simulink model "plant2016_cybership_detectabl_switching_bumplessExperiment"  (R2015b)
settings: Solver=VariableStepAuto  SolverMode=SingleTasking  StartTime=0.0  StopTime=150  FixedStep=.01  RelTol=1e-3  AbsTol=1e-6
StartFcn:
  | %plot_Contr_index('open')
libraries: simulink x9
(part 1 of 2)
CloseFcn:
  | ;slview('closediagram',bdroot);
settings Model: ExtModeTrigMode=oneshot  ExtModeArmWhenConnect=off  Creator=mjun  LastModifiedBy=TordFO
settings DataIOCC: LimitDataPoints=off  SaveFormat=Array  SignalLoggingSaveFormat=ModelDataLogs  SaveOutput=off  SaveTime=off
settings OptimizationCC: BlockReduction=off  BooleanDataType=off
settings DebuggingCC: SaveWithParameterizedLinksMsg=none  UnderspecifiedInitializationDetection=Classic  MergeDetectMultiDrivingBlocksExec=none  SignalResolutionControl=TryResolveAllWithWarning  MultiTaskDSMMsg=warning  MultiTaskCondExecSysMsg=none
settings HardwareCC: ProdBitPerPointer=32  ProdLargestAtomicFloat=None  ProdIntDivRoundTo=Undefined  ProdEndianess=Unspecified  ProdWordSize=32  ProdHWDeviceType=32-bit Generic  TargetUnknown=on
settings RTWCC: TemplateMakefile=grt_unix.tmf
settings GRTTargetCC: GeneratePreprocessorConditionals=Disable all  CombineOutputUpdateFcns=off  GRTInterface=on
settings ConfigComp: CovModelRefEnable=Off  CovSFcnEnable=off

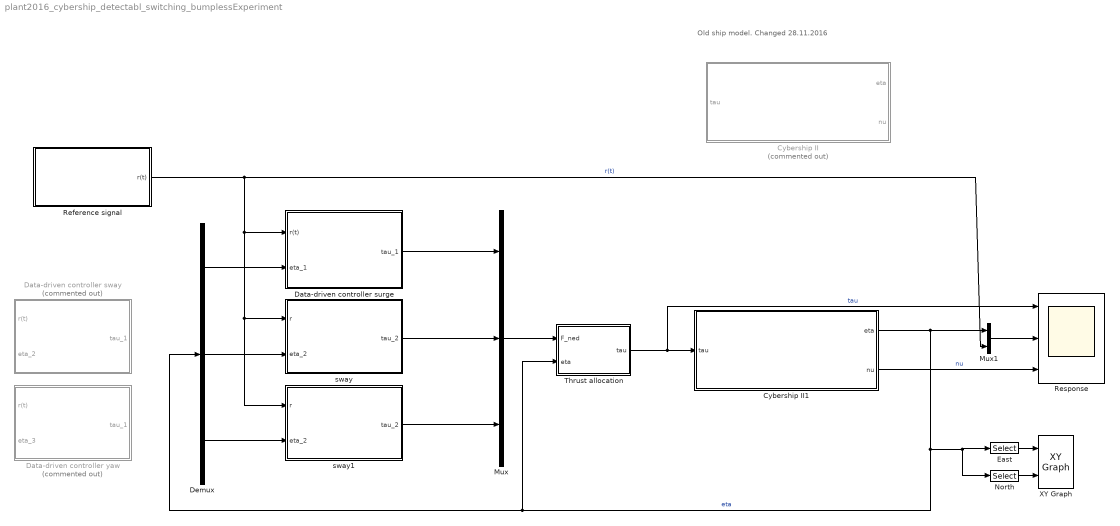
== system plant2016_cybership_detectabl_switching_bumplessExperiment ==
  note: Old ship model. Changed 28.11.2016
  Cybership II : Subsystem  Commented=on  mask{eta_0=[1;2;20*pi/180], nu_0=[0;0;0], first_order_waves_on_off=off, wind_on_off=off, surge_only=off}
      mask prompts: eta_0 "Position initial state"; nu_0 "Velocity initial state"; first_order_waves_on_off "First order wave disturbances"; wind_on_off "Wind loads"; surge_only "Only surge"
      mask Display: image('CybershipIII.jpg')
  Cybership II1 : Subsystem  mask{eta_0=[0;0;0], nu_0=[0;0;0], surge_only=off, first_order_waves_on_off=off, wind_on_off=on, rand_wind=off, wind_dir=180+45}
      mask prompts: eta_0 "Position initial state"; nu_0 "Velocity initial state"; surge_only "Only surge"; first_order_waves_on_off "First order wave disturbances"; wind_on_off "Wind loads"; rand_wind "Random wind direction"
      mask DialogControl Container9 Prompt: Forces
      mask DialogControl Control2 Prompt: Wind Direction [0,360):
      mask Display: image('CybershipIII.jpg')
  Data-driven controller surge : Subsystem
  Data-driven controller sway : Subsystem  Commented=on
  Data-driven controller yaw : Subsystem  Commented=on
  Demux : Demux  Outputs=3
  East : Selector  InputPortWidth=3  IndexOptions=Index vector (dialog)  Indices=[2]  OutputSizes=1
  Mux : Mux  Inputs=3
  Mux1 : Mux  Inputs=2
  North : Selector  InputPortWidth=3  IndexOptions=Index vector (dialog)  Indices=[1]  OutputSizes=1
  Reference signal : Subsystem
  Response : Scope  NumInputPorts=3
  Thrust allocation : Subsystem  mask(Thrust allocation block){surge_control_on_off=on, sway_control_on_off=on, yaw_control_on_off=on}
      mask prompts: surge_control_on_off "Surge Thrust on"; sway_control_on_off "Sway Thrust on"; yaw_control_on_off "Yaw Thrust on"
      mask help: Thrust allocation block. The block rotates the NED-force vector to the body frame where the ship is actuated in pure surge, sway and yaw. Any of the thrust direction can be enabeled/disabeled, but note that reference tracking is only possible for both surge and sway thrust enabeled.
  XY Graph : simulink/Sinks/XY Graph  xmin=-1  xmax=1  ymin=-1  ymax=1  st=-1
  sway : Subsystem  mask{sway_Kp=2, sway_Ki=0.1, sway_Kd=10}
      mask prompts: sway_Kp "Kp"; sway_Ki "Ki"; sway_Kd "Kd"
  sway1 : Subsystem  mask{yaw_Kp=2, yaw_Ki=0.3, yaw_Kd=2}
      mask prompts: yaw_Kp "Kp"; yaw_Ki "Ki"; yaw_Kd "Kd"
  wires:
  Reference signal/1(r(t)) -> Mux1/2, sway1/1(r), sway/1(r), Data-driven controller surge/1(r(t))  "r(t)"
  Cybership II1/2(nu) -> Response/3  "nu"
  Demux/3 -> sway1/2(eta_2)
  Demux/1 -> Data-driven controller surge/2(eta_1)
  Mux1/1 -> Response/2
  North/1 -> XY Graph/2
  East/1 -> XY Graph/1
  Demux/2 -> sway/2(eta_2)
  Cybership II1/1(eta) -> Mux1/1, North/1, East/1, Thrust allocation/2(eta), Demux/1  "eta"
  Data-driven controller surge/1(tau_1) -> Mux/1
  Thrust allocation/1(tau) -> Cybership II1/1(tau), Response/1  "tau"
  Mux/1 -> Thrust allocation/1(F_ned)
  sway/1(tau_2) -> Mux/2
  sway1/1(tau_2) -> Mux/3

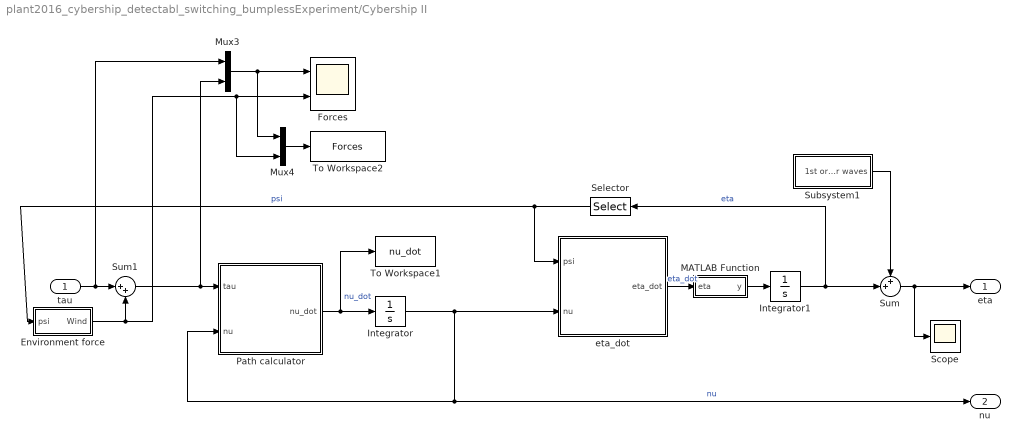
== system plant2016_cybership_detectabl_switching_bumplessExperiment/Cybership II ==
  tau : Inport
  Environment force : Subsystem
  Forces : Scope  NumInputPorts=2
  Integrator : Integrator  InitialCondition=nu_0
  Integrator1 : Integrator  InitialCondition=eta_0
  MATLAB Function : MATLAB Function  TreatAsAtomicUnit=on
  Mux3 : Mux  Inputs=2
  Mux4 : Mux  Inputs=2
  Path calculator : MATLAB Function  TreatAsAtomicUnit=on
  Scope : Scope
  Selector : Selector  InputPortWidth=3  IndexOptions=Index vector (dialog)  Indices=3  OutputSizes=1
  Subsystem1 : Subsystem
  Sum : Sum  Inputs=++|
  Sum1 : Sum  Inputs=|++
  To Workspace1 : ToWorkspace  VariableName=nu_dot  SaveFormat=Timeseries  SampleTime=-1
  To Workspace2 : ToWorkspace  VariableName=Forces  SaveFormat=Timeseries  SampleTime=-1
  eta_dot : MATLAB Function  TreatAsAtomicUnit=on
  eta : Outport
  nu : Outport  Port=2
  wires:
  Sum1/1 -> Mux3/2, Path calculator/1(tau)
  eta_dot/1(eta_dot) -> MATLAB Function/1(eta)  "eta_dot"
  Path calculator/1(nu_dot) -> To Workspace1/1, Integrator/1  "nu_dot"
  Integrator1/1 -> Sum/2, Selector/1  "eta"
  Integrator/1 -> nu/1, Path calculator/2(nu), eta_dot/2(nu)  "nu"
  Selector/1 -> eta_dot/1(psi), Environment force/1(psi)  "psi"
  MATLAB Function/1(y) -> Integrator1/1
  Sum/1 -> Scope/1, eta/1
  Subsystem1/1(1st order waves) -> Sum/1
  tau/1 -> Mux3/1, Sum1/1
  Environment force/1(Wind) -> Mux4/2, Forces/2, Sum1/2
  Mux3/1 -> Mux4/1, Forces/1
  Mux4/1 -> To Workspace2/1

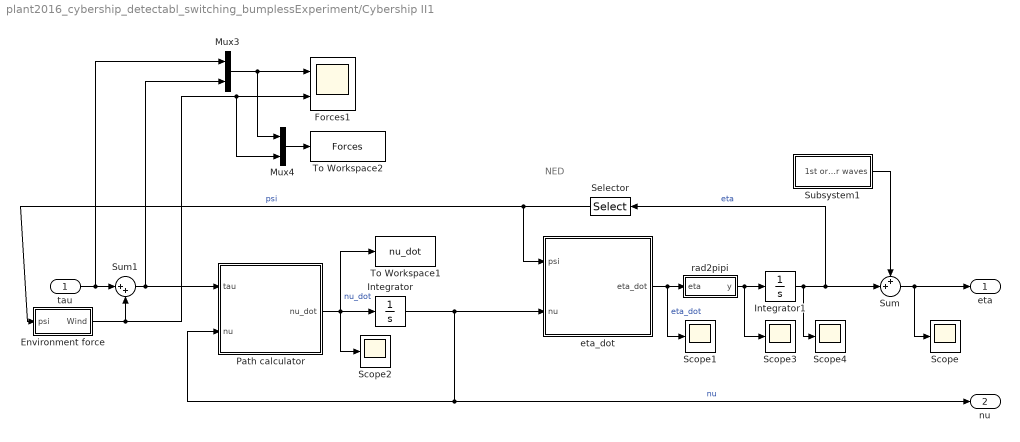
== system plant2016_cybership_detectabl_switching_bumplessExperiment/Cybership II1 ==
  note: NED
  tau : Inport
  Environment force : Subsystem
  Forces1 : Scope  NumInputPorts=2
  Integrator : Integrator  InitialCondition=nu_0
  Integrator1 : Integrator  InitialCondition=eta_0
  Mux3 : Mux  Inputs=2
  Mux4 : Mux  Inputs=2
  Path calculator : MATLAB Function  TreatAsAtomicUnit=on
  Scope{,1..4} (5 alike) : Scope
  Selector : Selector  InputPortWidth=3  IndexOptions=Index vector (dialog)  Indices=3  OutputSizes=1
  Subsystem1 : Subsystem
  Sum : Sum  Inputs=++|
  Sum1 : Sum  Inputs=|++
  To Workspace1 : ToWorkspace  VariableName=nu_dot  SaveFormat=Timeseries  SampleTime=-1
  To Workspace2 : ToWorkspace  VariableName=Forces  SaveFormat=Timeseries  SampleTime=-1
  eta_dot : MATLAB Function  TreatAsAtomicUnit=on
  rad2pipi : MATLAB Function  TreatAsAtomicUnit=on
  eta : Outport
  nu : Outport  Port=2
  wires:
  Sum1/1 -> Mux3/2, Path calculator/1(tau)
  eta_dot/1(eta_dot) -> Scope1/1, rad2pipi/1(eta)  "eta_dot"
  Path calculator/1(nu_dot) -> Scope2/1, To Workspace1/1, Integrator/1  "nu_dot"
  Integrator1/1 -> Scope4/1, Sum/2, Selector/1  "eta"
  Integrator/1 -> nu/1, Path calculator/2(nu), eta_dot/2(nu)  "nu"
  Selector/1 -> eta_dot/1(psi), Environment force/1(psi)  "psi"
  rad2pipi/1(y) -> Scope3/1, Integrator1/1
  Sum/1 -> Scope/1, eta/1
  Subsystem1/1(1st order waves) -> Sum/1
  tau/1 -> Mux3/1, Sum1/1
  Environment force/1(Wind) -> Forces1/2, Mux4/2, Sum1/2
  Mux3/1 -> Forces1/1, Mux4/1
  Mux4/1 -> To Workspace2/1

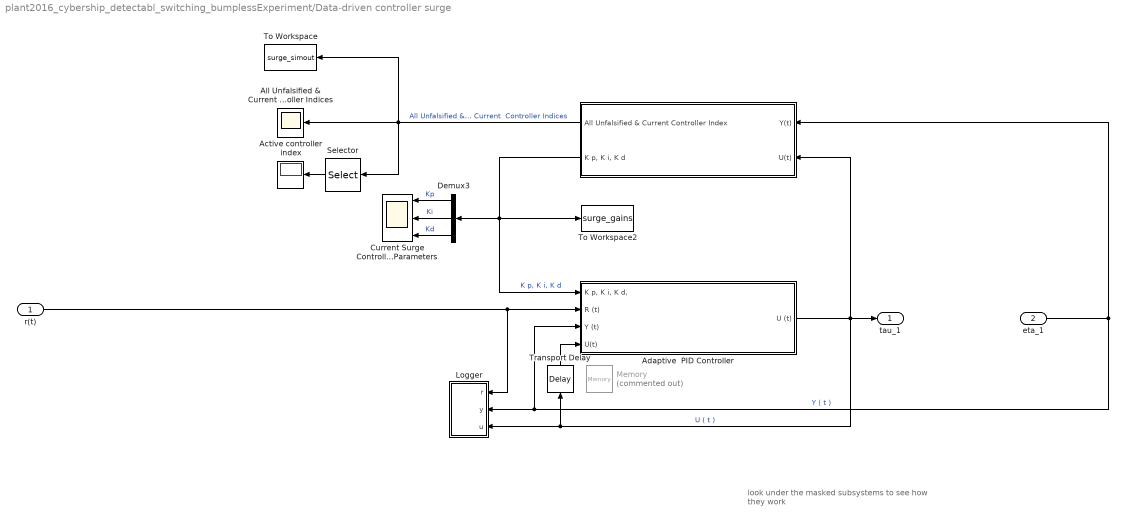
== system plant2016_cybership_detectabl_switching_bumplessExperiment/Data-driven controller surge ==
  note: look under the masked subsystems
      |  to see how they work
  r(t) : Inport
  eta_1 : Inport  Port=2
  " " : Subsystem  Priority=1  mask(Unfalsification Algorithm){w1_n=1.*[1 20], w1_d=2*[1 3], w2_n=0.01, w2_d=1.2*[1 3 3 1], C_p=[3], C_i=[1], C_d=[10], rho=0.5}
      mask prompts: w1_n "Numerater of filter W1"; w1_d "Denominater of filter W1"; w2_n "Numerater of filter W2"; w2_d "Denominater of filter W2"; C_p "Set of proportional gains, (horizontal vector)"; C_i "Set of integral gains, (horizontal vector)"; C_d "Set of derivative gains, (horizontal vector)"; rho "Set Hysteresis switching limit"
      mask help:
      | Look under the mask see how "Unfalsification Algorithm" works.
      |
      | Initially, from U & Y, the S-function "fic_ref" generates online the ficticious reference signal for all Candidate Controllers. The S-function "cost_func" then calculates the cost/ performance index for each candidate controllers. Then, based on these Performance Indices, the unfalsification algorithm selects the optimal controller for every instant and outputs the controller parameter ( in our case which is the value of Kp, Ki, Kd).
      |
      | The initilization command of this block calls a m-file "initilization". This m-file sets the port size of the mux & demux blocks inside the subsystem to the number of initial candidate controller whenever the user changes the set of initial condidate controller from the parameter entry block of this subsystem.
      |
      | Original filter-parameters:
      | w1_num =   [1 20]
      | w1_dem = 2*[1 3]
      | w2_num = 0.01
      | w2_den = 1.2*[1 3 3 1]
      mask init:
      | surge_initialization
      mask Help:
      | Look under the mask see how "Unfalsification Algorithm" works.
      | Initially, from U & Y, the S-function "fic_ref" generates online the ficticious reference signal for all Candidate Controllers.
      | The S-function "cost_func" then calculates the cost/ performance index for each candidate controllers.
      | Then, based on these Performance Indices, the S-Function "Supervisor.m" selects the optimal controller for every instant and outputs the controller parameter ( in our case which is the value of Kp, Ki, Kd).
      | The initilization command of this block calls a m-file "initilization". This m-file sets the port size of the mux & demux blocks inside the subsystem to the number of initial candidate controller whenever the user changes the set of initial condidate controller from the parameter entry block of this subsystem.
      mask Display: disp('Unfalsification Algorithm')
  Active controller index : Display
  Adaptive  PID Controller : Subsystem  mask(Adaptive PID Controller){Epsilon=0.1, Delta=0.01}
      mask prompts: Delta "Sampling time"
      mask init:
      | global epsilon delta
      | epsilon=Epsilon; delta = Delta;
      mask Help: This is an Adaptive PID Controller subsystem. The PID controller parameter (Kp, Ki, Kd) is determined at each instant by the Unfalsification algorithm. Look under the mask to see how this block works. The initilization commands of this block declares "epsilon" & "delta" as global variables. "epsilon" is the time-constant for approximate derivative and "delta" is the sampling time for all s-functions. Other S-functions under the Unfalsification Subsystem access these 2 variables by declaring them as global in their respective m-files.
      mask Display: disp('Adaptive PID Controller')
  All Unfalsified & Current Controller Indices : Scope
      settings: Tag=cont_plot
  Current Surge Controller Parameters : Scope  NumInputPorts=3
  Demux3 : Demux  Outputs=3
  Logger : Subsystem
  Memory : Memory  Commented=on
  Selector : Selector  IndexOptions=Index vector (dialog)  Indices=[1]  OutputSizes=1
  To Workspace : ToWorkspace  VariableName=surge_simout  SaveFormat=Timeseries  SampleTime=-1
  To Workspace2 : ToWorkspace  VariableName=surge_gains  SaveFormat=Timeseries  SampleTime=-1
  Transport Delay : TransportDelay  DelayTime=0.01
  tau_1 : Outport
  wires:
  " "/1(All Unfalsified & Current Controller Index) -> To Workspace/1, All Unfalsified & Current Controller Indices/1, Selector/1  "All Unfalsified & Current  Controller Indices"
  Adaptive  PID Controller/1(U (t)) -> tau_1/1, Transport Delay/1, Logger/3(u), " "/2(U(t))  "U ( t )"
  " "/2("K p, K i, K d") -> Adaptive  PID Controller/1("K p, K i, K d,"), To Workspace2/1, Demux3/1  "K p, K i, K d"
  eta_1/1 -> " "/1(Y(t)), Logger/2(y), Adaptive  PID Controller/3(Y (t))  "Y ( t )"
  Demux3/1 -> Current Surge Controller Parameters/1  "Kp"
  r(t)/1 -> Logger/1(r), Adaptive  PID Controller/2(R (t))
  Demux3/2 -> Current Surge Controller Parameters/2  "Ki"
  Demux3/3 -> Current Surge Controller Parameters/3  "Kd"
  Selector/1 -> Active controller index/1
  Transport Delay/1 -> Adaptive  PID Controller/4(U(t))

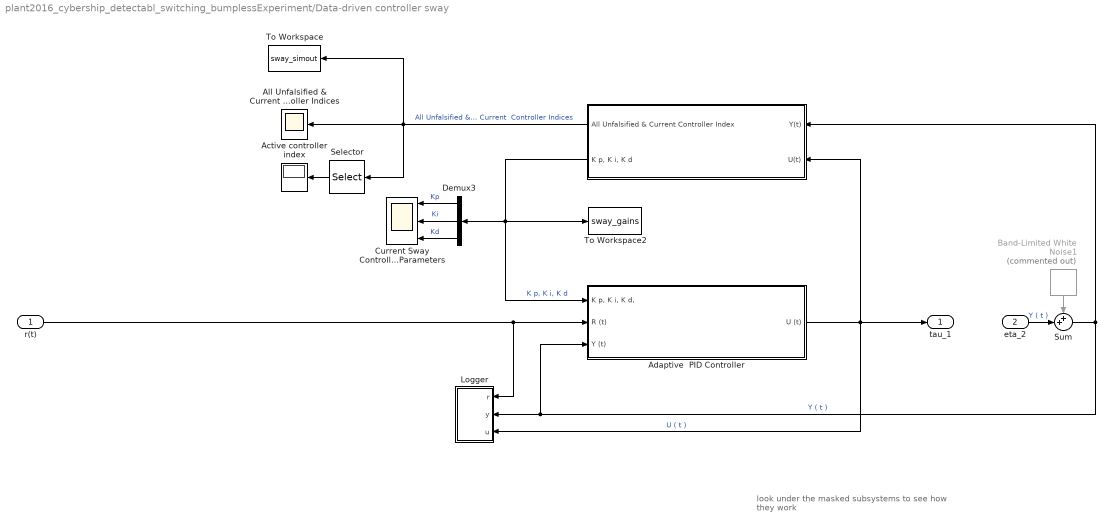
== system plant2016_cybership_detectabl_switching_bumplessExperiment/Data-driven controller sway ==
  note: look under the masked subsystems
      |  to see how they work
  r(t) : Inport
  eta_2 : Inport  Port=2
  " " : Subsystem  Priority=1  mask(Unfalsification Algorithm){w1_n=1.*[1 20], w1_d=2*[1 3], w2_n=0.01, w2_d=1.2*[1 3 3 1], C_p=2, C_i=0.1, C_d=10, rho=0}
      mask prompts: w1_n "Numerater of filter W1"; w1_d "Denominater of filter W1"; w2_n "Numerater of filter W2"; w2_d "Denominater of filter W2"; C_p "Set of proportional gains, (horizontal vector)"; C_i "Set of integral gains, (horizontal vector)"; C_d "Set of derivative gains, (horizontal vector)"; rho "Set cost-limit"
      mask help:
      | Look under the mask see how "Unfalsification Algorithm" works.
      |
      | Initially, from U & Y, the S-function "fic_ref" generates online the ficticious reference signal for all Candidate Controllers. The S-function "cost_func" then calculates the cost/ performance index for each candidate controllers. Then, based on these Performance Indices, the unfalsification algorithm selects the optimal controller for every instant and outputs the controller parameter ( in our case which is the value of Kp, Ki, Kd).
      |
      | The initilization command of this block calls a m-file "initilization". This m-file sets the port size of the mux & demux blocks inside the subsystem to the number of initial candidate controller whenever the user changes the set of initial condidate controller from the parameter entry block of this subsystem.
      |
      | Original filter-parameters:
      | w1_num =   [1 20]
      | w1_dem = 2*[1 3]
      | w2_num = 0.01
      | w2_den = 1.2*[1 3 3 1]
      mask init:
      | sway_initialization
      mask Help:
      | Look under the mask see how "Unfalsification Algorithm" works.
      | Initially, from U & Y, the S-function "fic_ref" generates online the ficticious reference signal for all Candidate Controllers.
      | The S-function "cost_func" then calculates the cost/ performance index for each candidate controllers.
      | Then, based on these Performance Indices, the S-Function "Supervisor.m" selects the optimal controller for every instant and outputs the controller parameter ( in our case which is the value of Kp, Ki, Kd).
      | The initilization command of this block calls a m-file "initilization". This m-file sets the port size of the mux & demux blocks inside the subsystem to the number of initial candidate controller whenever the user changes the set of initial condidate controller from the parameter entry block of this subsystem.
      mask Display: disp('Unfalsification Algorithm')
  Active controller index : Display
  Adaptive  PID Controller : Subsystem  mask(Adaptive PID Controller){Epsilon=.01, Delta=.01}
      mask prompts: Delta "Sampling time"
      mask init:
      | global epsilon delta
      | epsilon=Epsilon; delta = Delta;
      mask Help: This is an Adaptive PID Controller subsystem. The PID controller parameter (Kp, Ki, Kd) is determined at each instant by the Unfalsification algorithm. Look under the mask to see how this block works. The initilization commands of this block declares "epsilon" & "delta" as global variables. "epsilon" is the time-constant for approximate derivative and "delta" is the sampling time for all s-functions. Other S-functions under the Unfalsification Subsystem access these 2 variables by declaring them as global in their respective m-files.
      mask Display: disp('Adaptive PID Controller')
  All Unfalsified & Current Controller Indices : Scope
      settings: Tag=cont_plot
  Band-Limited White Noise1 : simulink/Sources/Band-Limited White Noise  Commented=on  Cov=[0.00001]  Ts=0.01  seed=[23341]
  Current Sway Controller Parameters : Scope  NumInputPorts=3
  Demux3 : Demux  Outputs=3
  Logger : Subsystem
  Selector : Selector  IndexOptions=Index vector (dialog)  Indices=[1]  OutputSizes=1
  Sum : Sum  Inputs=++|
  To Workspace : ToWorkspace  VariableName=sway_simout  SaveFormat=Timeseries  SampleTime=-1
  To Workspace2 : ToWorkspace  VariableName=sway_gains  SaveFormat=Timeseries  SampleTime=-1
  tau_1 : Outport
  wires:
  Selector/1 -> Active controller index/1
  Demux3/3 -> Current Sway Controller Parameters/3  "Kd"
  Band-Limited White Noise1/1 -> Sum/1
  Demux3/2 -> Current Sway Controller Parameters/2  "Ki"
  eta_2/1 -> Sum/2  "Y ( t )"
  r(t)/1 -> Logger/1(r), Adaptive  PID Controller/2(R (t))
  Demux3/1 -> Current Sway Controller Parameters/1  "Kp"
  Sum/1 -> " "/1(Y(t)), Adaptive  PID Controller/3(Y (t)), Logger/2(y)  "Y ( t )"
  " "/2("K p, K i, K d") -> Demux3/1, To Workspace2/1, Adaptive  PID Controller/1("K p, K i, K d,")  "K p, K i, K d"
  Adaptive  PID Controller/1(U (t)) -> tau_1/1, " "/2(U(t)), Logger/3(u)  "U ( t )"
  " "/1(All Unfalsified & Current Controller Index) -> Selector/1, All Unfalsified & Current Controller Indices/1, To Workspace/1  "All Unfalsified & Current  Controller Indices"

== system plant2016_cybership_detectabl_switching_bumplessExperiment/Data-driven controller yaw ==
  note: look under the masked subsystems
      |  to see how they work
  r(t) : Inport
  eta_3 : Inport  Port=2
  " " : Subsystem  Priority=1  mask(Unfalsification Algorithm){w1_n=1.*[1 20], w1_d=2*[1 3], w2_n=0.01, w2_d=1.2*[1 3 3 1], C_p=2, C_i=0.3, C_d=2, rho=0}
      mask prompts: w1_n "Numerater of filter W1"; w1_d "Denominater of filter W1"; w2_n "Numerater of filter W2"; w2_d "Denominater of filter W2"; C_p "Set of proportional gains, (horizontal vector)"; C_i "Set of integral gains, (horizontal vector)"; C_d "Set of derivative gains, (horizontal vector)"; rho "Set cost-limit"
      mask help:
      | Look under the mask see how "Unfalsification Algorithm" works.
      |
      | Initially, from U & Y, the S-function "fic_ref" generates online the ficticious reference signal for all Candidate Controllers. The S-function "cost_func" then calculates the cost/ performance index for each candidate controllers. Then, based on these Performance Indices, the unfalsification algorithm selects the optimal controller for every instant and outputs the controller parameter ( in our case which is the value of Kp, Ki, Kd).
      |
      | The initilization command of this block calls a m-file "initilization". This m-file sets the port size of the mux & demux blocks inside the subsystem to the number of initial candidate controller whenever the user changes the set of initial condidate controller from the parameter entry block of this subsystem.
      |
      | Original filter-parameters:
      | w1_num =   [1 20]
      | w1_dem = 2*[1 3]
      | w2_num = 0.01
      | w2_den = 1.2*[1 3 3 1]
      mask init:
      | yaw_initialization
      mask Help:
      | Look under the mask see how "Unfalsification Algorithm" works.
      | Initially, from U & Y, the S-function "fic_ref" generates online the ficticious reference signal for all Candidate Controllers.
      | The S-function "cost_func" then calculates the cost/ performance index for each candidate controllers.
      | Then, based on these Performance Indices, the S-Function "Supervisor.m" selects the optimal controller for every instant and outputs the controller parameter ( in our case which is the value of Kp, Ki, Kd).
      | The initilization command of this block calls a m-file "initilization". This m-file sets the port size of the mux & demux blocks inside the subsystem to the number of initial candidate controller whenever the user changes the set of initial condidate controller from the parameter entry block of this subsystem.
      mask Display: disp('Unfalsification Algorithm')
  Active controller index : Display
  Adaptive  PID Controller : Subsystem  mask(Adaptive PID Controller){Epsilon=.01, Delta=.01}
      mask prompts: Delta "Sampling time"
      mask init:
      | global epsilon delta
      | epsilon=Epsilon; delta = Delta;
      mask Help: This is an Adaptive PID Controller subsystem. The PID controller parameter (Kp, Ki, Kd) is determined at each instant by the Unfalsification algorithm. Look under the mask to see how this block works. The initilization commands of this block declares "epsilon" & "delta" as global variables. "epsilon" is the time-constant for approximate derivative and "delta" is the sampling time for all s-functions. Other S-functions under the Unfalsification Subsystem access these 2 variables by declaring them as global in their respective m-files.
      mask Display: disp('Adaptive PID Controller')
  All Unfalsified & Current Controller Indices : Scope
      settings: Tag=cont_plot
  Band-Limited White Noise1 : simulink/Sources/Band-Limited White Noise  Commented=on  Cov=[0.00001]  Ts=0.01  seed=[23341]
  Current Yaw Controller Parameters : Scope  NumInputPorts=3
  Demux3 : Demux  Outputs=3
  Logger : Subsystem
  Selector : Selector  IndexOptions=Index vector (dialog)  Indices=[1]  OutputSizes=1
  Sum : Sum  Inputs=++|
  To Workspace : ToWorkspace  VariableName=yaw_simout  SaveFormat=Timeseries  SampleTime=-1
  To Workspace2 : ToWorkspace  VariableName=yaw_gains  SaveFormat=Timeseries  SampleTime=-1
  tau_1 : Outport
  wires:
  " "/1(All Unfalsified & Current Controller Index) -> To Workspace/1, All Unfalsified & Current Controller Indices/1, Selector/1  "All Unfalsified & Current  Controller Indices"
  Adaptive  PID Controller/1(U (t)) -> Logger/3(u), tau_1/1, " "/2(U(t))  "U ( t )"
  " "/2("K p, K i, K d") -> Adaptive  PID Controller/1("K p, K i, K d,"), To Workspace2/1, Demux3/1  "K p, K i, K d"
  Sum/1 -> Logger/2(y), Adaptive  PID Controller/3(Y (t)), " "/1(Y(t))  "Y ( t )"
  Demux3/1 -> Current Yaw Controller Parameters/1  "Kp"
  r(t)/1 -> Adaptive  PID Controller/2(R (t)), Logger/1(r)
  eta_3/1 -> Sum/2  "Y ( t )"
  Demux3/2 -> Current Yaw Controller Parameters/2  "Ki"
  Band-Limited White Noise1/1 -> Sum/1
  Demux3/3 -> Current Yaw Controller Parameters/3  "Kd"
  Selector/1 -> Active controller index/1

== system plant2016_cybership_detectabl_switching_bumplessExperiment/Reference signal ==
  2nd order LP omega_n=0.1 : TransferFcn  Numerator=0.1^2  Denominator=[1 2*1*0.1 0.1^2]
  2nd order LP omega_n=0.2 : TransferFcn  Numerator=0.2^2  Denominator=[1 2*1*0.2 0.2^2]
  2nd order LP omega_n=0.33 : TransferFcn  Numerator=0.33^2  Denominator=[1 2*1*0.33 0.33^2]
  2nd order LP omega_n=0.4 : TransferFcn  Commented=through  Numerator=0.5^2  Denominator=[1 2*1*0.5 0.5^2]
  Add : Sum  Inputs=+++
  Constant : Constant  Value=4
  Constant1 : Constant  Value=0
  Manual Switch : ManualSwitch  CurrentSetting=0
  Multiport Switch : MultiPortSwitch  Inputs=4
  Step1 : Step  Time=5  SampleTime=0
  Step2 : Step  Time=30  SampleTime=0
  Step3 : Step  Time=60  After=-2  SampleTime=0
  r(t) : Outport
  wires:
  Add/1 -> 2nd order LP omega_n=0.1/1, 2nd order LP omega_n=0.2/1, 2nd order LP omega_n=0.33/1, 2nd order LP omega_n=0.4/1  "R ( t )"
  Multiport Switch/1 -> Manual Switch/1
  2nd order LP omega_n=0.1/1 -> Multiport Switch/2
  2nd order LP omega_n=0.2/1 -> Multiport Switch/3
  2nd order LP omega_n=0.33/1 -> Multiport Switch/4
  Step1/1 -> Add/1  "R ( t )"
  Step2/1 -> Add/2
  Step3/1 -> Add/3
  2nd order LP omega_n=0.4/1 -> Multiport Switch/5
  Constant/1 -> Multiport Switch/1
  Manual Switch/1 -> r(t)/1
  Constant1/1 -> Manual Switch/2

== system plant2016_cybership_detectabl_switching_bumplessExperiment/Thrust allocation ==
  F_ned : Inport
  eta : Inport  Port=2
  Demux1 : Demux  Outputs=3
  Mux2 : Mux  Inputs=3
  NED2b : MATLAB Function  TreatAsAtomicUnit=on
  Saturation : Saturate  UpperLimit=[3;3;3]  LowerLimit=[-3;-3;-3]
  Selector : Selector  InputPortWidth=3  IndexOptions=Index vector (dialog)  Indices=[3]  OutputSizes=1
  surge only : Subsystem
  sway only : Subsystem
  yaw only : Subsystem
  tau : Outport
  wires:
  Mux2/1 -> Saturation/1  "tau"
  Selector/1 -> NED2b/2(psi)
  F_ned/1 -> NED2b/1(tau)
  NED2b/1(tau_b) -> Demux1/1
  Demux1/3 -> yaw only/1(In1)
  yaw only/1(Out1) -> Mux2/3
  surge only/1(Out1) -> Mux2/1
  Demux1/2 -> sway only/1(In1)
  sway only/1(Out1) -> Mux2/2
  Demux1/1 -> surge only/1(In1)
  eta/1 -> Selector/1
  Saturation/1 -> tau/1

== system plant2016_cybership_detectabl_switching_bumplessExperiment/sway ==
  r : Inport
  eta_2 : Inport  Port=2
  Add : Sum  Inputs=++-
  Approximate Derivative : Subsystem  mask{sway_epsilon=0.01}
      mask prompts: sway_epsilon "Sway Epsilon"
  Gain : Gain  Gain=sway_Kp
  Gain1 : Gain  Gain=sway_Ki
  Gain2 : Gain  Gain=sway_Kd
  Integrator : Integrator
  Sum : Sum  Inputs=|+-
  tau_2 : Outport
  wires:
  Approximate Derivative/1(Out) -> Gain2/1
  Gain/1 -> Add/1
  Integrator/1 -> Gain1/1
  Gain2/1 -> Add/3
  Sum/1 -> Integrator/1, Gain/1
  Add/1 -> tau_2/1
  eta_2/1 -> Sum/2, Approximate Derivative/1(Y (t))
  Gain1/1 -> Add/2
  r/1 -> Sum/1

== system plant2016_cybership_detectabl_switching_bumplessExperiment/sway1 ==
  r : Inport
  eta_2 : Inport  Port=2
  Add : Sum  Inputs=++-
  Approximate Derivative : Subsystem  mask{yaw_epsilon=0.01}
      mask prompts: yaw_epsilon "Sway Epsilon"
  Gain : Gain  Gain=yaw_Kp
  Gain1 : Gain  Gain=yaw_Ki
  Gain2 : Gain  Gain=yaw_Kd
  Integrator : Integrator
  Sum : Sum  Inputs=|+-
  tau_2 : Outport
  wires:
  r/1 -> Sum/1
  Gain1/1 -> Add/2
  eta_2/1 -> Approximate Derivative/1(Y (t)), Sum/2
  Add/1 -> tau_2/1
  Sum/1 -> Gain/1, Integrator/1
  Gain2/1 -> Add/3
  Integrator/1 -> Gain1/1
  Gain/1 -> Add/1
  Approximate Derivative/1(Out) -> Gain2/1

== system plant2016_cybership_detectabl_switching_bumplessExperiment/Cybership II/Environment force ==
  psi : Inport
  All Wind forces : Scope
  Constant : Constant  Value=[0;0;0]
  Constant1 : Constant  Value=wind_on_off
  Constant2 : Constant  Value=surge_only
  Environment force1 : Subsystem
  Gain : Gain  Gain=[1;0;0]
  Switch : Switch  Criteria=u2 ~= 0
  Switch1 : Switch  Criteria=u2 ~= 0
  Wind : Outport
  wires:
  psi/1 -> Environment force1/1(psi)
  Switch/1 -> Switch1/3, Gain/1
  Constant/1 -> Switch/3
  Constant1/1 -> Switch/2
  Environment force1/1(Env. force) -> Switch/1
  Switch1/1 -> Wind/1, All Wind forces/1
  Gain/1 -> Switch1/1
  Constant2/1 -> Switch1/2

== system plant2016_cybership_detectabl_switching_bumplessExperiment/Cybership II/Subsystem1 ==
  1st order Wave motions : Scope
  Constant : Constant  Value=[0;0;0]
  Constant1 : Constant  Value=first_order_waves_on_off
  Constant2 : Constant  Value=surge_only
  Gain : Gain  Gain=[1;0;0]
  Subsystem : Subsystem  mask{start_time=0, omega_01=0.1, zeta_01=0.01, omega_02=0.1, zeta_02=0.1, omega_03=0.01, zeta_03=0.04}
      mask prompts: start_time "Wave start time"; omega_01 "Surge Dominating - wave frequency"; zeta_01 "Surge - Damping ratio"; omega_02 "Sway - Dominating wave frequency"; zeta_02 "Sway - Damping ratio"; omega_03 "Yaw - Dominating wave frequency"; zeta_03 "Yaw - Damping ratio"
      mask Display: disp('1st order Waves')
  Switch : Switch  Criteria=u2 ~= 0
  Switch1 : Switch  Criteria=u2 ~= 0
  1st order waves : Outport
  wires:
  Constant/1 -> Switch/3
  Constant1/1 -> Switch/2
  Subsystem/1(1st order waves) -> Switch/1
  Switch/1 -> Switch1/3, Gain/1
  Switch1/1 -> 1st order waves/1, 1st order Wave motions/1
  Gain/1 -> Switch1/1
  Constant2/1 -> Switch1/2

== system plant2016_cybership_detectabl_switching_bumplessExperiment/Cybership II1/Environment force ==
  psi : Inport
  All Wind forces : Scope
  Constant : Constant  Value=[0;0;0]
  Constant1 : Constant  Value=wind_on_off
  Constant2 : Constant  Value=surge_only
  Environment force1 : Subsystem
  Gain : Gain  Gain=[1;0;0]
  Switch : Switch  Criteria=u2 ~= 0
  Switch1 : Switch  Criteria=u2 ~= 0
  Wind : Outport
  wires:
  psi/1 -> Environment force1/1(psi)
  Switch/1 -> Switch1/3, Gain/1
  Constant/1 -> Switch/3
  Constant1/1 -> Switch/2
  Environment force1/1(Env. force) -> Switch/1
  Switch1/1 -> Wind/1, All Wind forces/1
  Gain/1 -> Switch1/1
  Constant2/1 -> Switch1/2

== system plant2016_cybership_detectabl_switching_bumplessExperiment/Cybership II1/Subsystem1 ==
  1st order Wave motions : Scope
  Constant : Constant  Value=[0;0;0]
  Constant1 : Constant  Value=first_order_waves_on_off
  Constant2 : Constant  Value=surge_only
  Gain : Gain  Gain=[1;0;0]
  Subsystem : Subsystem  mask{start_time=0, omega_01=0.6, zeta_01=0.01, omega_02=0.6, zeta_02=0.1, omega_03=0.01, zeta_03=0.04}
      mask prompts: start_time "Wave start time"; omega_01 "Surge Dominating - wave frequency"; zeta_01 "Surge - Damping ratio"; omega_02 "Sway - Dominating wave frequency"; zeta_02 "Sway - Damping ratio"; omega_03 "Yaw - Dominating wave frequency"; zeta_03 "Yaw - Damping ratio"
      mask Display: disp('1st order Waves')
  Switch : Switch  Criteria=u2 ~= 0
  Switch1 : Switch  Criteria=u2 ~= 0
  1st order waves : Outport
  wires:
  Constant/1 -> Switch/3
  Constant1/1 -> Switch/2
  Subsystem/1(1st order waves) -> Switch/1
  Switch/1 -> Switch1/3, Gain/1
  Switch1/1 -> 1st order waves/1, 1st order Wave motions/1
  Gain/1 -> Switch1/1
  Constant2/1 -> Switch1/2

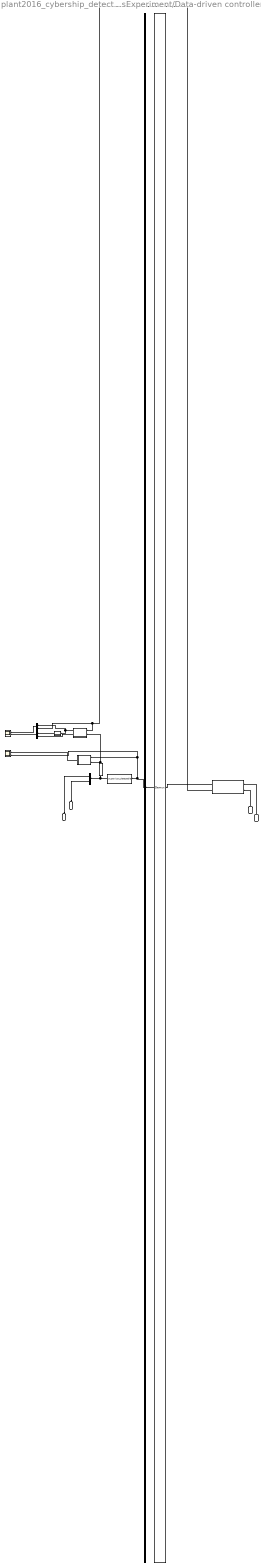
== system plant2016_cybership_detectabl_switching_bumplessExperiment/Data-driven controller surge/  ==
  note: Performance
      | Index of each
      | Candidate Controller
      | J (n)
  note: n - Candidate Controller Index
  Y(t) : Inport
  U(t) : Inport  Port=2
  Controller Selector : S-Function  FunctionName=Supervisor_detectable  Parameters=C_p, C_i, C_d, rho  SFunctionDeploymentMode=off  EnableBusSupport=off
  Cost Surge : Scope  NumInputPorts=2
  Demux. : Demux  Outputs=[3 -1]
  Demux1 : Demux  Tag=surge_demux_1  Outputs=1
  FRS Surge : Scope  NumInputPorts=2
  MATLAB Function : MATLAB Function  TreatAsAtomicUnit=on
  MATLAB Function1 : MATLAB Function  TreatAsAtomicUnit=on
  MATLAB Function2 : MATLAB Function  TreatAsAtomicUnit=on
  Mux : Mux  Inputs=2
  Mux1 : Mux  Tag=surge_mux_1  Inputs=1
  Mux2 : Mux  Inputs=2
  Selector : MATLAB Function  TreatAsAtomicUnit=on
  look under the subsystem to see how it works : Subsystem  Tag=surge_per_monitor
      mask Display: disp('Performance Monitor')
  All Unfalsified & Current Controller Index : Outport  InitialOutput=0
  "K p, K i, K d" : Outport  Port=2  InitialOutput=0
  wires:
  Demux./1 -> "K p, K i, K d"/1  "Current Controller Parameters"
  Demux./2 -> All Unfalsified & Current Controller Index/1
  Mux1/1 -> Controller Selector/1, Cost Surge/2, MATLAB Function/1(cost)  "Cost"
  look under the subsystem to see how it works/1(Out1) -> Demux1/1  "Performance Index of each candidate controller (n x 1)"
  Y(t)/1 -> look under the subsystem to see how it works/1(Y (t))
  U(t)/1 -> look under the subsystem to see how it works/2(U (t))
  Controller Selector/1 -> Demux./1, Selector/1(u)
  Selector/1(y) -> MATLAB Function1/2(i), MATLAB Function/2(i)
  MATLAB Function/1(y) -> Cost Surge/1  "Current"
  look under the subsystem to see how it works/2(frs) -> MATLAB Function1/1(frs), Mux/2  "FRS"
  MATLAB Function1/1(y) -> MATLAB Function2/1(u), Mux/1  "Current"
  MATLAB Function1/2(y_sqr) -> Mux2/2  "FRS_squared"
  Mux/1 -> FRS Surge/1
  Mux2/1 -> FRS Surge/2
  MATLAB Function2/1(y) -> Mux2/1  "Current"
  Demux1/1 -> Mux1/1

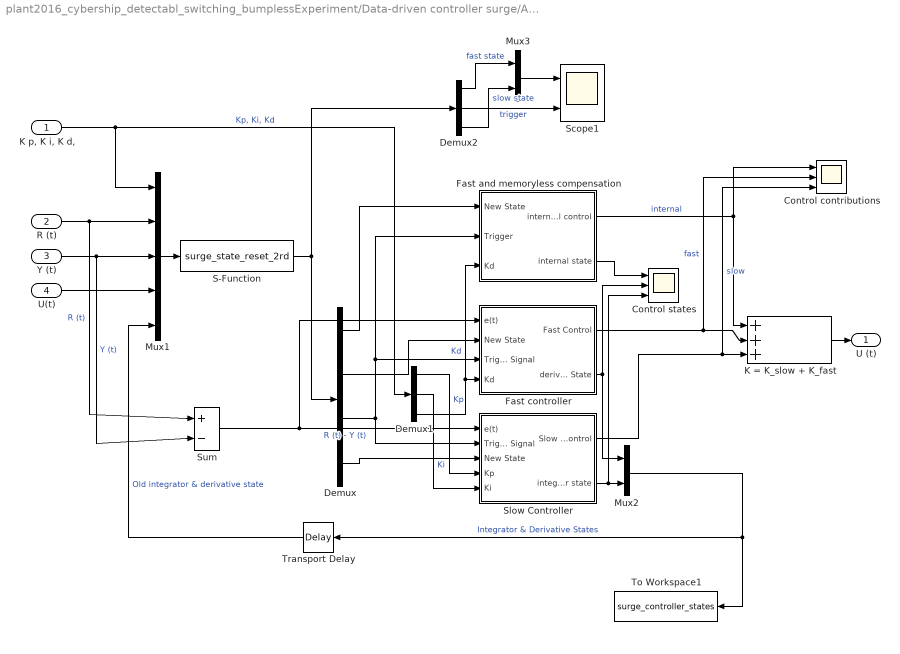
== system plant2016_cybership_detectabl_switching_bumplessExperiment/Data-driven controller surge/Adaptive  PID Controller ==
  "K p, K i, K d," : Inport
  R (t) : Inport  Port=2
  Y (t) : Inport  Port=3
  U(t) : Inport  Port=4
  Control contributions : Scope  NumInputPorts=3
  Control states : Scope  NumInputPorts=3
  Demux : Demux
  Demux1 : Demux  Outputs=3
  Demux2 : Demux  Outputs=3
  Fast and memoryless compensation : Subsystem  mask{A=-1, C=1}
  Fast controller : Subsystem
  K = K_slow + K_fast : Sum  Inputs=+++
  Mux1 : Mux  Inputs=5
  Mux2 : Mux  Inputs=2
  Mux3 : Mux  Inputs=2
  S-Function : S-Function  FunctionName=surge_state_reset_2rd  Parameters=epsilon, delta  SFunctionDeploymentMode=off  EnableBusSupport=off
  Scope1 : Scope  NumInputPorts=2
  Slow Controller : Subsystem
  "Sum " : Sum  Inputs=+|-  SaturateOnIntegerOverflow=on  InputSameDT=on  OutDataTypeStr=Inherit: Same as first input
  To Workspace1 : ToWorkspace  VariableName=surge_controller_states  SaveFormat=Timeseries  SampleTime=-1
  Transport Delay : TransportDelay  DelayTime=delta  InitialOutput=[0;0]
  U (t) : Outport  InitialOutput=0
  wires:
  Fast controller/2(derivative State) -> Control states/2, Mux2/1
  S-Function/1 -> Demux2/1, Demux/1
  Mux1/1 -> S-Function/1
  R (t)/1 -> "Sum "/1, Mux1/2  "R (t)"
  "K p, K i, K d,"/1 -> Mux1/1, Demux1/1  "Kp, Ki, Kd"
  Mux2/1 -> Transport Delay/1, To Workspace1/1  "Integrator & Derivative States"
  Transport Delay/1 -> Mux1/5  "Old integrator & derivative state"
  Y (t)/1 -> "Sum "/2, Mux1/3  "Y (t)"
  U(t)/1 -> Mux1/4
  Slow Controller/2(integrator state) -> Control states/3, Mux2/2
  "Sum "/1 -> Fast controller/1(e(t)), Slow Controller/1(e(t))  "R (t) - Y (t)"
  Demux/2 -> Fast controller/2(New State)
  Demux/4 -> Slow Controller/3(New State)
  Demux/3 -> Fast and memoryless compensation/2(Trigger), Fast controller/3(Trigger Signal), Slow Controller/2(Trigger Signal)
  Demux1/1 -> Slow Controller/4(Kp)  "Kp"
  Demux1/2 -> Slow Controller/5(Ki)  "Ki"
  Demux1/3 -> Fast and memoryless compensation/3(Kd), Fast controller/4(Kd)  "Kd"
  Slow Controller/1(Slow Control) -> K = K_slow + K_fast/3, Control contributions/3  "slow"
  Fast controller/1(Fast Control) -> Control contributions/2, K = K_slow + K_fast/2  "fast"
  K = K_slow + K_fast/1 -> U (t)/1
  Demux2/1 -> Mux3/1  "fast state"
  Demux2/2 -> Scope1/2  "trigger"
  Demux2/3 -> Mux3/2  "slow state"
  Mux3/1 -> Scope1/1
  Demux/1 -> Fast and memoryless compensation/1(New State)
  Fast and memoryless compensation/1(internal control) -> Control contributions/1, K = K_slow + K_fast/1  "internal"
  Fast and memoryless compensation/2(internal state) -> Control states/1

== system plant2016_cybership_detectabl_switching_bumplessExperiment/Data-driven controller surge/Logger ==
  r : Inport
  y : Inport  Port=2
  u : Inport  Port=3
  Mux1 : Mux
  Subtract : Sum  Inputs=+-
  To Workspace1 : ToWorkspace  VariableName=surge_result  SaveFormat=Timeseries  SampleTime=-1
  wires:
  Mux1/1 -> To Workspace1/1
  Subtract/1 -> Mux1/3  "e"
  u/1 -> Mux1/4  "u"
  r/1 -> Mux1/1, Subtract/2  "r"
  y/1 -> Mux1/2, Subtract/1  "y"

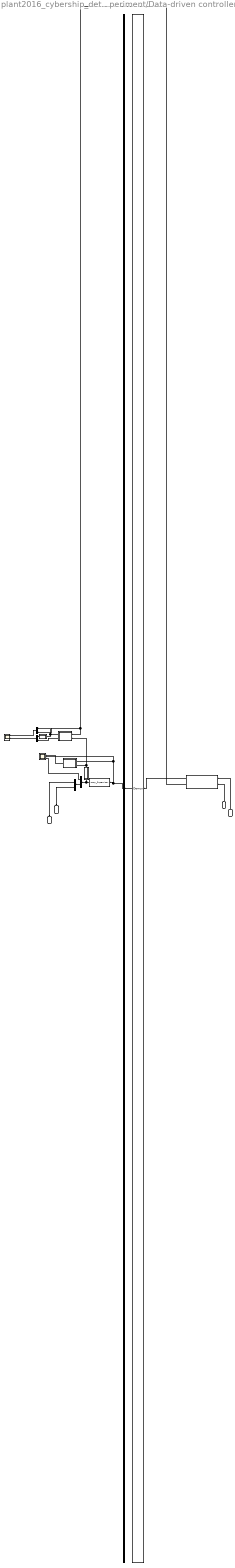
== system plant2016_cybership_detectabl_switching_bumplessExperiment/Data-driven controller sway/  ==
  note: n - Candidate Controller Index
  note: Performance
      | Index of each
      | Candidate Controller
      | J (n)
  Y(t) : Inport
  U(t) : Inport  Port=2
  Controller Selector : S-Function  FunctionName=sway_Supervisor  Parameters=C_p, C_i, C_d, rho  SFunctionDeploymentMode=off  EnableBusSupport=off
  Cost Sway : Scope  NumInputPorts=3
  Demux. : Demux  Outputs=[3 -1]
  Demux.1 : Demux  Outputs=[1 -1]
  Demux1 : Demux  Tag=sway_demux_1  Outputs=1
  FRS Sway : Scope  NumInputPorts=2
  MATLAB Function : MATLAB Function  TreatAsAtomicUnit=on
  MATLAB Function1 : MATLAB Function  TreatAsAtomicUnit=on
  MATLAB Function2 : MATLAB Function  TreatAsAtomicUnit=on
  Mux : Mux  Inputs=2
  Mux1 : Mux  Tag=sway_mux_1  Inputs=1
  Mux2 : Mux  Inputs=2
  Selector : MATLAB Function  TreatAsAtomicUnit=on
  look under the subsystem to see how it works : Subsystem  Tag=sway_per_monitor
      mask Display: disp('Performance Monitor')
  All Unfalsified & Current Controller Index : Outport  InitialOutput=0
  "K p, K i, K d" : Outport  Port=2  InitialOutput=0
  wires:
  MATLAB Function2/1(y) -> Mux2/1
  Mux2/1 -> FRS Sway/2  "FRS squared"
  Mux/1 -> FRS Sway/1  "FRS"
  MATLAB Function1/2(y_sqr) -> Mux2/2
  MATLAB Function1/1(y) -> MATLAB Function2/1(u), Mux/1
  look under the subsystem to see how it works/2(frs) -> MATLAB Function1/1(frs), Mux/2
  MATLAB Function/1(y) -> Cost Sway/1
  Selector/1(y) -> MATLAB Function/2(i), MATLAB Function1/2(i)
  Demux.1/1 -> Cost Sway/3  "rho"
  Demux.1/2 -> Demux./1
  U(t)/1 -> look under the subsystem to see how it works/2(U (t))
  Y(t)/1 -> look under the subsystem to see how it works/1(Y (t))
  look under the subsystem to see how it works/1(Out1) -> Demux1/1  "Performance Index of each candidate controller (n x 1)"
  Mux1/1 -> Controller Selector/1, Cost Sway/2, MATLAB Function/1(cost)  "(n x 1)"
  Demux./2 -> All Unfalsified & Current Controller Index/1
  Demux./1 -> "K p, K i, K d"/1  "Current Controller Parameters"
  Controller Selector/1 -> Demux.1/1, Selector/1(u)
  Demux1/1 -> Mux1/1

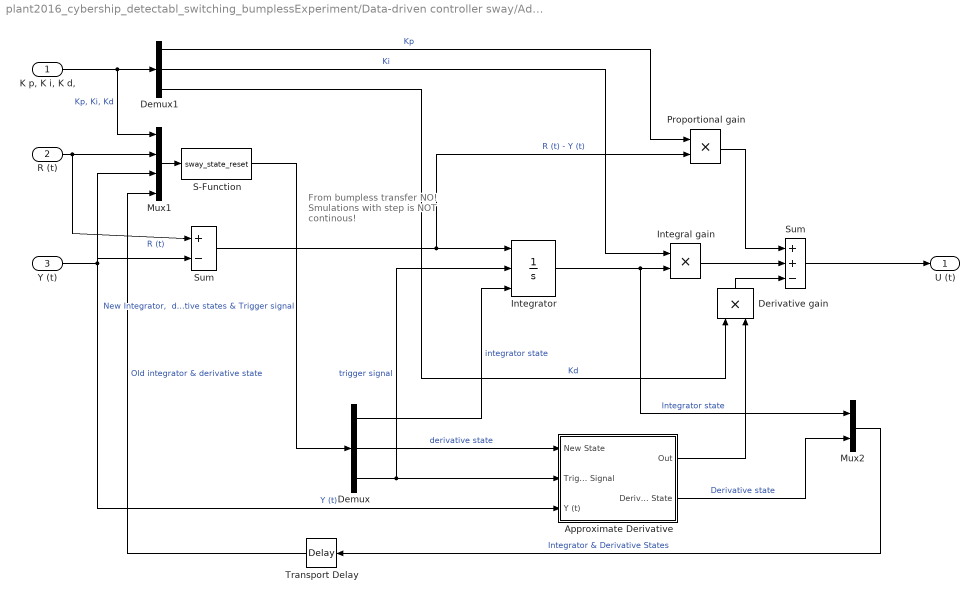
== system plant2016_cybership_detectabl_switching_bumplessExperiment/Data-driven controller sway/Adaptive  PID Controller ==
  note: From bumpless transfer
      | NO! Smulations
      | with step is NOT
      | continous!
  "K p, K i, K d," : Inport
  R (t) : Inport  Port=2
  Y (t) : Inport  Port=3
  Approximate Derivative : Subsystem
  Demux : Demux  Outputs=3
  Demux1 : Demux  Outputs=3
  Derivative gain : Product  SaturateOnIntegerOverflow=on  RndMeth=Zero  InputSameDT=on  OutDataTypeStr=Inherit: Same as first input
  Integral gain : Product  SaturateOnIntegerOverflow=on  RndMeth=Zero  InputSameDT=on  OutDataTypeStr=Inherit: Same as first input
  Integrator : Integrator  ExternalReset=either  InitialConditionSource=external
  Mux1 : Mux
  Mux2 : Mux  Inputs=2
  Proportional gain : Product  SaturateOnIntegerOverflow=on  RndMeth=Zero  InputSameDT=on  OutDataTypeStr=Inherit: Same as first input
  S-Function : S-Function  FunctionName=sway_state_reset  Parameters=epsilon, delta  SFunctionDeploymentMode=off  EnableBusSupport=off
      mask Help:
      | S function, inside "Adaptive PID Controller" block, for resetting the
      | controller state, when switching to a new controller, in order to reduce unwanted abrupt peaks in control signal u(t). Also generates trigger signal for the same purpose.
  Sum : Sum  Inputs=++-  SaturateOnIntegerOverflow=on  InputSameDT=on  OutDataTypeStr=Inherit: Same as first input
  "Sum " : Sum  Inputs=+|-  SaturateOnIntegerOverflow=on  InputSameDT=on  OutDataTypeStr=Inherit: Same as first input
  Transport Delay : TransportDelay  DelayTime=delta
  U (t) : Outport  InitialOutput=0
  wires:
  Y (t)/1 -> Approximate Derivative/3(Y (t)), Mux1/3, "Sum "/2  "Y (t)"
  Demux/3 -> Approximate Derivative/2(Trigger Signal), Integrator/2  "trigger signal"
  Transport Delay/1 -> Mux1/4  "Old integrator & derivative state"
  Mux2/1 -> Transport Delay/1  "Integrator & Derivative States"
  "K p, K i, K d,"/1 -> Demux1/1, Mux1/1  "Kp, Ki, Kd"
  R (t)/1 -> "Sum "/1, Mux1/2  "R (t)"
  Mux1/1 -> S-Function/1
  S-Function/1 -> Demux/1  "New Integrator,  derivative states & Trigger signal"
  Demux1/3 -> Derivative gain/1  "Kd"
  Demux/2 -> Approximate Derivative/1(New State)  "derivative state"
  Approximate Derivative/2(Derivative State) -> Mux2/2  "Derivative state"
  Demux/1 -> Integrator/3  "integrator state"
  Demux1/1 -> Proportional gain/1  "Kp"
  Demux1/2 -> Integral gain/1  "Ki"
  Sum/1 -> U (t)/1
  "Sum "/1 -> Proportional gain/2, Integrator/1  "R (t) - Y (t)"
  Integrator/1 -> Mux2/1, Integral gain/2  "Integrator state"
  Derivative gain/1 -> Sum/3
  Integral gain/1 -> Sum/2
  Approximate Derivative/1(Out) -> Derivative gain/2
  Proportional gain/1 -> Sum/1

== system plant2016_cybership_detectabl_switching_bumplessExperiment/Data-driven controller sway/Logger ==
  r : Inport
  y : Inport  Port=2
  u : Inport  Port=3
  Mux1 : Mux
  Subtract : Sum  Inputs=+-
  To Workspace1 : ToWorkspace  VariableName=sway_result  SaveFormat=Timeseries  SampleTime=-1
  wires:
  y/1 -> Subtract/1, Mux1/2  "y"
  r/1 -> Subtract/2, Mux1/1  "r"
  u/1 -> Mux1/4  "u"
  Subtract/1 -> Mux1/3  "e"
  Mux1/1 -> To Workspace1/1

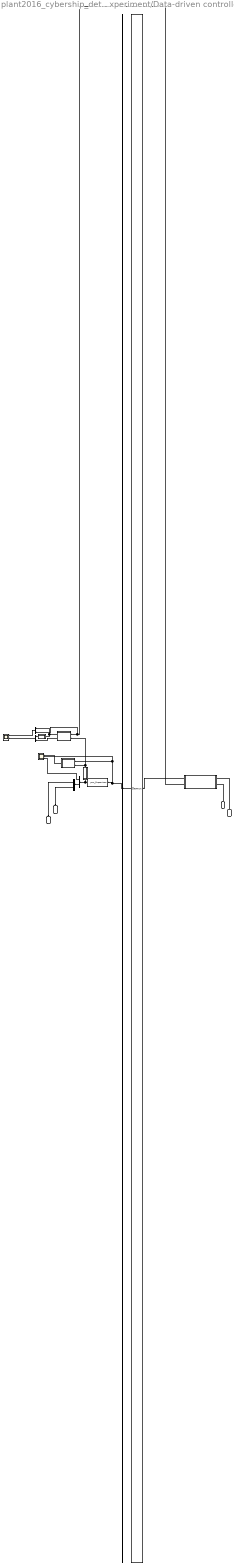
== system plant2016_cybership_detectabl_switching_bumplessExperiment/Data-driven controller yaw/  ==
  note: Performance
      | Index of each
      | Candidate Controller
      | J (n)
  note: n - Candidate Controller Index
  Y(t) : Inport
  U(t) : Inport  Port=2
  Controller Selector : S-Function  FunctionName=yaw_Supervisor  Parameters=C_p, C_i, C_d, rho  SFunctionDeploymentMode=off  EnableBusSupport=off
  Cost : Scope  NumInputPorts=3
  Demux. : Demux  Outputs=[3 -1]
  Demux.1 : Demux  Outputs=[1 -1]
  Demux1 : Demux  Tag=yaw_demux_1  Outputs=1
  FRS : Scope  NumInputPorts=2
  MATLAB Function : MATLAB Function  TreatAsAtomicUnit=on
  MATLAB Function1 : MATLAB Function  TreatAsAtomicUnit=on
  MATLAB Function2 : MATLAB Function  TreatAsAtomicUnit=on
  Mux : Mux  Inputs=2
  Mux1 : Mux  Tag=yaw_mux_1  Inputs=1
  Mux2 : Mux  Inputs=2
  Selector : MATLAB Function  TreatAsAtomicUnit=on
  look under the subsystem to see how it works : Subsystem  Tag=yaw_per_monitor
      mask Display: disp('Performance Monitor')
  All Unfalsified & Current Controller Index : Outport  InitialOutput=0
  "K p, K i, K d" : Outport  Port=2  InitialOutput=0
  wires:
  Controller Selector/1 -> Selector/1(u), Demux.1/1
  Demux./1 -> "K p, K i, K d"/1  "Current Controller Parameters"
  Demux./2 -> All Unfalsified & Current Controller Index/1
  Mux1/1 -> Cost/2, MATLAB Function/1(cost), Controller Selector/1  "(n x 1)"
  look under the subsystem to see how it works/1(Out1) -> Demux1/1  "Performance Index of each candidate controller (n x 1)"
  Y(t)/1 -> look under the subsystem to see how it works/1(Y (t))
  U(t)/1 -> look under the subsystem to see how it works/2(U (t))
  Demux.1/2 -> Demux./1
  Demux.1/1 -> Cost/3  "rho"
  Selector/1(y) -> MATLAB Function1/2(i), MATLAB Function/2(i)
  MATLAB Function/1(y) -> Cost/1
  look under the subsystem to see how it works/2(frs) -> Mux/2, MATLAB Function1/1(frs)
  MATLAB Function1/1(y) -> MATLAB Function2/1(u), Mux/1
  MATLAB Function1/2(y_sqr) -> Mux2/2
  Mux/1 -> FRS/1  "FRS"
  Mux2/1 -> FRS/2  "FRS squared"
  MATLAB Function2/1(y) -> Mux2/1
  Demux1/1 -> Mux1/1

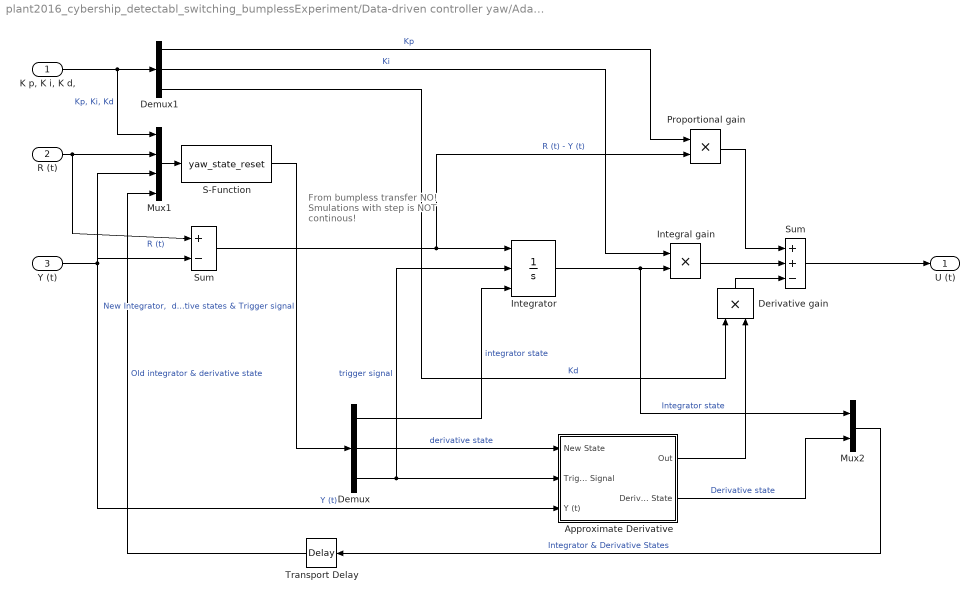
== system plant2016_cybership_detectabl_switching_bumplessExperiment/Data-driven controller yaw/Adaptive  PID Controller ==
  note: From bumpless transfer
      | NO! Smulations
      | with step is NOT
      | continous!
  "K p, K i, K d," : Inport
  R (t) : Inport  Port=2
  Y (t) : Inport  Port=3
  Approximate Derivative : Subsystem
  Demux : Demux  Outputs=3
  Demux1 : Demux  Outputs=3
  Derivative gain : Product  SaturateOnIntegerOverflow=on  RndMeth=Zero  InputSameDT=on  OutDataTypeStr=Inherit: Same as first input
  Integral gain : Product  SaturateOnIntegerOverflow=on  RndMeth=Zero  InputSameDT=on  OutDataTypeStr=Inherit: Same as first input
  Integrator : Integrator  ExternalReset=either  InitialConditionSource=external
  Mux1 : Mux
  Mux2 : Mux  Inputs=2
  Proportional gain : Product  SaturateOnIntegerOverflow=on  RndMeth=Zero  InputSameDT=on  OutDataTypeStr=Inherit: Same as first input
  S-Function : S-Function  FunctionName=yaw_state_reset  Parameters=epsilon, delta  SFunctionDeploymentMode=off  EnableBusSupport=off
      mask Help:
      | S function, inside "Adaptive PID Controller" block, for resetting the
      | controller state, when switching to a new controller, in order to reduce unwanted abrupt peaks in control signal u(t). Also generates trigger signal for the same purpose.
  Sum : Sum  Inputs=++-  SaturateOnIntegerOverflow=on  InputSameDT=on  OutDataTypeStr=Inherit: Same as first input
  "Sum " : Sum  Inputs=+|-  SaturateOnIntegerOverflow=on  InputSameDT=on  OutDataTypeStr=Inherit: Same as first input
  Transport Delay : TransportDelay  DelayTime=delta
  U (t) : Outport  InitialOutput=0
  wires:
  Proportional gain/1 -> Sum/1
  Approximate Derivative/1(Out) -> Derivative gain/2
  Integral gain/1 -> Sum/2
  Derivative gain/1 -> Sum/3
  Integrator/1 -> Integral gain/2, Mux2/1  "Integrator state"
  "Sum "/1 -> Integrator/1, Proportional gain/2  "R (t) - Y (t)"
  Sum/1 -> U (t)/1
  Demux1/2 -> Integral gain/1  "Ki"
  Demux1/1 -> Proportional gain/1  "Kp"
  Demux/1 -> Integrator/3  "integrator state"
  Approximate Derivative/2(Derivative State) -> Mux2/2  "Derivative state"
  Demux/2 -> Approximate Derivative/1(New State)  "derivative state"
  Demux1/3 -> Derivative gain/1  "Kd"
  S-Function/1 -> Demux/1  "New Integrator,  derivative states & Trigger signal"
  Mux1/1 -> S-Function/1
  R (t)/1 -> Mux1/2, "Sum "/1  "R (t)"
  "K p, K i, K d,"/1 -> Mux1/1, Demux1/1  "Kp, Ki, Kd"
  Mux2/1 -> Transport Delay/1  "Integrator & Derivative States"
  Transport Delay/1 -> Mux1/4  "Old integrator & derivative state"
  Demux/3 -> Integrator/2, Approximate Derivative/2(Trigger Signal)  "trigger signal"
  Y (t)/1 -> "Sum "/2, Mux1/3, Approximate Derivative/3(Y (t))  "Y (t)"

== system plant2016_cybership_detectabl_switching_bumplessExperiment/Data-driven controller yaw/Logger ==
  r : Inport
  y : Inport  Port=2
  u : Inport  Port=3
  Mux1 : Mux
  Subtract : Sum  Inputs=+-
  To Workspace1 : ToWorkspace  VariableName=yaw_result  SaveFormat=Timeseries  SampleTime=-1
  wires:
  Mux1/1 -> To Workspace1/1
  Subtract/1 -> Mux1/3  "e"
  u/1 -> Mux1/4  "u"
  r/1 -> Mux1/1, Subtract/2  "r"
  y/1 -> Mux1/2, Subtract/1  "y"

== system plant2016_cybership_detectabl_switching_bumplessExperiment/Thrust allocation/surge only ==
  In1 : Inport
  Constant : Constant  Value=0
  Constant1 : Constant  Value=surge_control_on_off
  Switch : Switch  Criteria=u2 ~= 0
  Out1 : Outport
  wires:
  Constant1/1 -> Switch/2
  Constant/1 -> Switch/3
  In1/1 -> Switch/1
  Switch/1 -> Out1/1

== system plant2016_cybership_detectabl_switching_bumplessExperiment/Thrust allocation/sway only ==
  In1 : Inport
  Constant2 : Constant  Value=0
  Constant3 : Constant  Value=sway_control_on_off
  Switch1 : Switch  Criteria=u2 ~= 0
  Out1 : Outport
  wires:
  In1/1 -> Switch1/1
  Switch1/1 -> Out1/1
  Constant3/1 -> Switch1/2
  Constant2/1 -> Switch1/3

== system plant2016_cybership_detectabl_switching_bumplessExperiment/Thrust allocation/yaw only ==
  In1 : Inport
  Constant : Constant  Value=0
  Constant1 : Constant  Value=yaw_control_on_off
  Switch : Switch  Criteria=u2 ~= 0
  Out1 : Outport
  wires:
  In1/1 -> Switch/1
  Switch/1 -> Out1/1
  Constant/1 -> Switch/3
  Constant1/1 -> Switch/2

== system plant2016_cybership_detectabl_switching_bumplessExperiment/sway/Approximate Derivative ==
  Y (t) : Inport
  Gain : Gain  Gain=1/sway_epsilon^2  SaturateOnIntegerOverflow=on  OutDataTypeStr=Inherit: Same as input  ParamDataTypeStr=Inherit: Same as input
  Gain1 : Gain  Gain=1/sway_epsilon  SaturateOnIntegerOverflow=on  OutDataTypeStr=Inherit: Same as input  ParamDataTypeStr=Inherit: Same as input
  Gain2 : Gain  Gain=1/sway_epsilon  SaturateOnIntegerOverflow=on  OutDataTypeStr=Inherit: Same as input  ParamDataTypeStr=Inherit: Same as input
  Integrator : Integrator
  Sum : Sum  Inputs=+-  SaturateOnIntegerOverflow=on  InputSameDT=on  OutDataTypeStr=Inherit: Same as first input
  Sum1 : Sum  Inputs=+-  SaturateOnIntegerOverflow=on  InputSameDT=on  OutDataTypeStr=Inherit: Same as first input
  Out : Outport
  wires:
  Integrator/1 -> Gain/1, Gain2/1
  Gain/1 -> Sum1/2
  Sum1/1 -> Out/1
  Gain2/1 -> Sum/2
  Gain1/1 -> Sum1/1
  Y (t)/1 -> Sum/1, Gain1/1
  Sum/1 -> Integrator/1

== system plant2016_cybership_detectabl_switching_bumplessExperiment/sway1/Approximate Derivative ==
  Y (t) : Inport
  Gain : Gain  Gain=1/yaw_epsilon^2  SaturateOnIntegerOverflow=on  OutDataTypeStr=Inherit: Same as input  ParamDataTypeStr=Inherit: Same as input
  Gain1 : Gain  Gain=1/yaw_epsilon  SaturateOnIntegerOverflow=on  OutDataTypeStr=Inherit: Same as input  ParamDataTypeStr=Inherit: Same as input
  Gain2 : Gain  Gain=1/yaw_epsilon  SaturateOnIntegerOverflow=on  OutDataTypeStr=Inherit: Same as input  ParamDataTypeStr=Inherit: Same as input
  Integrator : Integrator
  Sum : Sum  Inputs=+-  SaturateOnIntegerOverflow=on  InputSameDT=on  OutDataTypeStr=Inherit: Same as first input
  Sum1 : Sum  Inputs=+-  SaturateOnIntegerOverflow=on  InputSameDT=on  OutDataTypeStr=Inherit: Same as first input
  Out : Outport
  wires:
  Sum/1 -> Integrator/1
  Y (t)/1 -> Gain1/1, Sum/1
  Gain1/1 -> Sum1/1
  Gain2/1 -> Sum/2
  Sum1/1 -> Out/1
  Gain/1 -> Sum1/2
  Integrator/1 -> Gain2/1, Gain/1

== system plant2016_cybership_detectabl_switching_bumplessExperiment/Cybership II/Environment force/Environment force1 ==
  psi : Inport
  Add : Sum  Inputs=2
  Mean wind : Subsystem  mask{windStrength=5, start=50}
      mask prompts: windStrength "Wind Strength"; start "Start Time"
  Scope : Scope
  Slowly varying : Subsystem  mask{start=70}
      mask prompts: start "Start Time"
  Wind direction : Subsystem
  Wind force : MATLAB Function  TreatAsAtomicUnit=on
  Wind-Scope : Scope
  r2d : Gain  Gain=180/pi
  Env. force : Outport
  wires:
  Add/1 -> Wind force/3(u)
  Wind force/1(y) -> Wind-Scope/1, Env. force/1
  psi/1 -> Wind force/2(psi)
  Wind direction/1(beta_w) -> r2d/1, Wind force/1(beta_w)
  r2d/1 -> Scope/1
  Mean wind/1(Mean wind) -> Add/1
  Slowly varying/1(Slowly varying) -> Add/2
